simulink model "Beamforming"  (R2019a)
settings: Solver=FixedStepAuto  StartTime=0.0  StopTime=10  RelTol=1e-3
undefined symbols (not defined in the file or in its folder): phased
libraries: dspstat3 x2, phasedtxrxlib x2, phaseddoalib x2
settings Model: Creator=saadn  LastModifiedBy=saadn
settings OptimizationCC: DefaultParameterBehavior=Inlined  UseDivisionForNetSlopeComputation=on  GainParamInheritBuiltInType=on  UseFloatMulNetSlope=on  InlineInvariantSignals=on  PassReuseOutputArgsAs=Individual arguments  ZeroExternalMemoryAtStartup=off  ZeroInternalMemoryAtStartup=off  NoFixptDivByZeroProtection=on  EfficientFloat2IntCast=on  LifeSpan=1  OptimizeBlockOrder=speed  DifferentSizesBufferReuse=on
settings DebuggingCC: ParameterTunabilityLossMsg=error
settings HardwareCC: ProdLongLongMode=on
settings SFSimCC: MATLABDynamicMemAlloc=off
settings RTWCC: SystemTargetFile=ert.tlc  GenCodeOnly=on  TemplateMakefile=ert_default_tmf  GenerateReport=on  IncludeHyperlinkInReport=on  LaunchReport=on  TargetLang=C++  GenerateTraceInfo=on  GenerateTraceReport=on  GenerateTraceReportSl=on  GenerateTraceReportSf=on  GenerateTraceReportEml=on
settings CodeAppCC: GenerateComments=off  IgnoreCustomStorageClasses=off  OperatorAnnotations=on  SimulinkDataObjDesc=on  SFDataObjDesc=on  CustomSymbolStrGlobalVar=rt$N$M  CustomSymbolStrType=$N$M  CustomSymbolStrFcn=$N$M$F  CustomSymbolStrMacro=$N$M  InsertBlockDesc=on
settings ERTTargetCC: TargetLangStandard=C++03 (ISO)  GenerateSampleERTMain=on  IncludeMdlTerminateFcn=off  CombineSignalStateStructs=on  MultiInstanceERTCode=on  CodeInterfacePackaging=C++ class  SupportContinuousTime=on  InlinedParameterPlacement=NonHierarchical  RootIOFormat=Structure reference  ERTCustomFileTemplate=example_file_process.tlc  ERTFilePackagingFormat=CompactWithDataFile

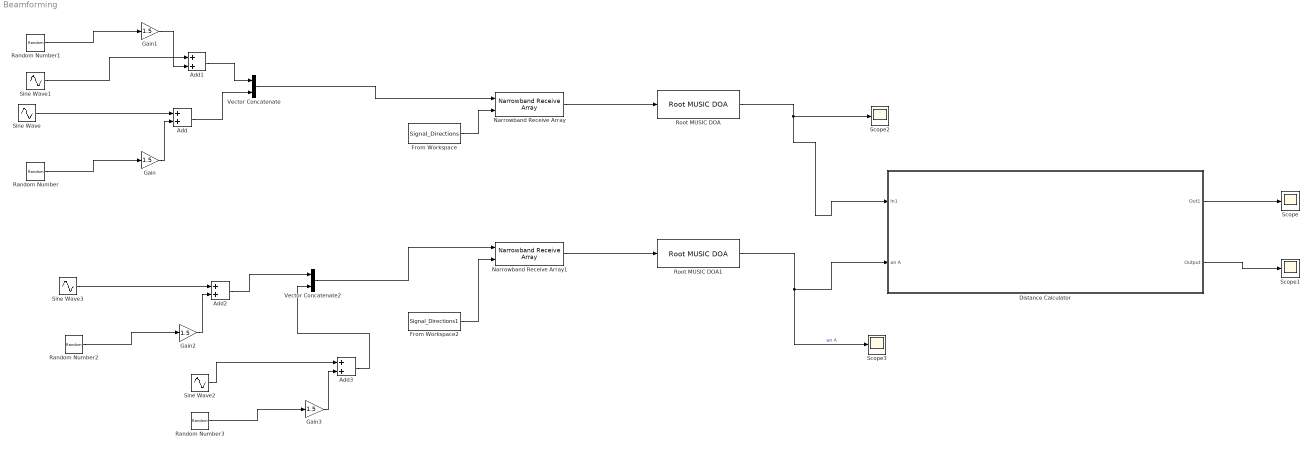
== system Beamforming ==
  Add{,1..3} (4 alike) : Sum
  "Distance Calculator " : Subsystem
  From Workspace : FromWorkspace  VariableName=Signal_Directions  SampleTime=1
  From Workspace2 : FromWorkspace  VariableName=Signal_Directions1  SampleTime=1
  Gain{,1..3} (4 alike) : Gain  Gain=1.5
  Narrowband Receive Array : phasedtxrxlib/Narrowband Receive Array  PropagationSpeed=343  OperatingFrequency=250  Wavefront=Plane  SensorGainMeasure=dB  Polarization=None  WeightsInputPort=off  SimulateUsing=Interpreted execution  Sensor=phased.ULA('Element',phased.IsotropicAntennaElement('FrequencyRange',[ 50, 500 ]),'NumElements',2,'ElementSpacing',0.1)
      settings: SourceProductName=Phased Array System Toolbox  SourceProductBaseCode=AR
  Narrowband Receive Array1 : phasedtxrxlib/Narrowband Receive Array  PropagationSpeed=343  OperatingFrequency=250  Wavefront=Plane  SensorGainMeasure=dB  Polarization=None  WeightsInputPort=off  SimulateUsing=Interpreted execution  Sensor=phased.ULA('Element',phased.IsotropicAntennaElement('FrequencyRange',[ 50, 500 ]),'NumElements',2,'ElementSpacing',0.1)
      settings: SourceProductName=Phased Array System Toolbox  SourceProductBaseCode=AR
  Random Number{,1..3} (4 alike) : RandomNumber  Variance=0.25  SampleTime=0
  Root MUSIC DOA : phaseddoalib/Root MUSIC DOA  PropagationSpeed=343  OperatingFrequency=250  NumSignalsSource=Property  NumSignalsMethod=AIC  NumSignals=1  ForwardBackwardAveraging=off  SpatialSmoothing=0  SimulateUsing=Interpreted execution  SensorArray=phased.ULA('Element',phased.IsotropicAntennaElement('FrequencyRange',[ 50, 500 ]),'NumElements',2,'ElementSpacing',0.1)
      settings: SourceProductName=Phased Array System Toolbox  SourceProductBaseCode=AR
  Root MUSIC DOA1 : phaseddoalib/Root MUSIC DOA  PropagationSpeed=343  OperatingFrequency=250  NumSignalsSource=Property  NumSignalsMethod=AIC  NumSignals=1  ForwardBackwardAveraging=off  SpatialSmoothing=0  SimulateUsing=Interpreted execution  SensorArray=phased.ULA('Element',phased.IsotropicAntennaElement('FrequencyRange',[ 50, 500 ]),'NumElements',2,'ElementSpacing',0.1)
      settings: SourceProductName=Phased Array System Toolbox  SourceProductBaseCode=AR
  Scope{,1..3} (4 alike) : Scope
  Sine Wave : Sin  Amplitude=0.8  Frequency=1067  SampleTime=0
  Sine Wave1 : Sin  Frequency=1067  SampleTime=0
  Sine Wave2 : Sin  Amplitude=0.7  Frequency=1067  SampleTime=0
  Sine Wave3 : Sin  Amplitude=0.8  Frequency=1067  SampleTime=0
  Vector Concatenate : Concatenate
  Vector Concatenate2 : Concatenate
  wires:
  From Workspace/1 -> Narrowband Receive Array/2
  Sine Wave1/1 -> Add1/1
  Sine Wave/1 -> Add/1
  Vector Concatenate2/1 -> Narrowband Receive Array1/1
  From Workspace2/1 -> Narrowband Receive Array1/2
  Root MUSIC DOA/1 -> "Distance Calculator "/1(In1), Scope2/1
  Root MUSIC DOA1/1 -> Scope3/1, "Distance Calculator "/2(an A)  "an A"
  "Distance Calculator "/1(Out1) -> Scope/1
  "Distance Calculator "/2(Output) -> Scope1/1
  Gain/1 -> Add/2
  Random Number/1 -> Gain/1
  Random Number1/1 -> Gain1/1
  Gain1/1 -> Add1/2
  Add/1 -> Vector Concatenate/2
  Add1/1 -> Vector Concatenate/1
  Vector Concatenate/1 -> Narrowband Receive Array/1
  Sine Wave3/1 -> Add2/1
  Random Number2/1 -> Gain2/1
  Gain2/1 -> Add2/2
  Add2/1 -> Vector Concatenate2/1
  Sine Wave2/1 -> Add3/1
  Random Number3/1 -> Gain3/1
  Gain3/1 -> Add3/2
  Add3/1 -> Vector Concatenate2/2
  Narrowband Receive Array/1 -> Root MUSIC DOA/1
  Narrowband Receive Array1/1 -> Root MUSIC DOA1/1

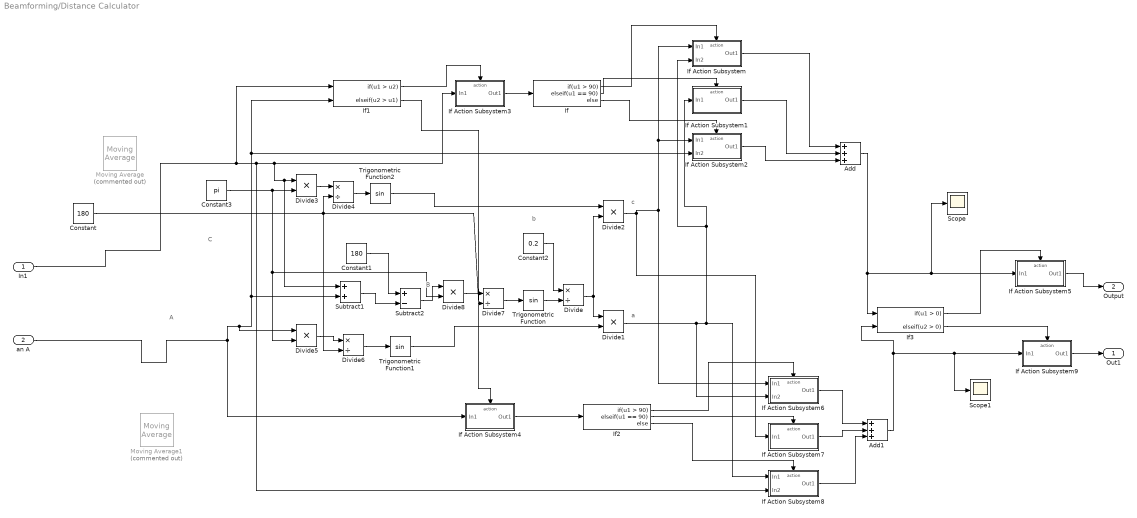
== system Beamforming/Distance Calculator  ==
  note: c
  note: b
  note: a
  note: B
  note: C
  note: A
  In1 : Inport
  an A : Inport  Port=2
  Add : Sum  Inputs=+++
  Add1 : Sum  Inputs=+++
  Constant : Constant  Value=180
  Constant1 : Constant  Value=180
  Constant2 : Constant  Value=0.2
  Constant3 : Constant  Value=pi
  Divide{,4,6..7} (4 alike) : Product  Inputs=*/
  Divide{1..3,5,8} (5 alike) : Product  Inputs=**
  If : If  IfExpression=u1 > 90  ElseIfExpressions=u1 == 90
  If Action Subsystem : Subsystem  TreatAsAtomicUnit=on
  If Action Subsystem1 : Subsystem  TreatAsAtomicUnit=on
  If Action Subsystem2 : Subsystem  TreatAsAtomicUnit=on
  If Action Subsystem3 : Subsystem  TreatAsAtomicUnit=on
  If Action Subsystem4 : Subsystem  TreatAsAtomicUnit=on
  If Action Subsystem5 : Subsystem  TreatAsAtomicUnit=on
  If Action Subsystem6 : Subsystem  TreatAsAtomicUnit=on
  If Action Subsystem7 : Subsystem  TreatAsAtomicUnit=on
  If Action Subsystem8 : Subsystem  TreatAsAtomicUnit=on
  If Action Subsystem9 : Subsystem  TreatAsAtomicUnit=on
  If1 : If  NumInputs=2  IfExpression=u1 > u2  ElseIfExpressions=u2 > u1  ShowElse=off
  If2 : If  IfExpression=u1 > 90  ElseIfExpressions=u1 == 90
  If3 : If  NumInputs=2  ElseIfExpressions=u2 > 0  ShowElse=off
  Moving Average : dspstat3/Moving Average  Commented=on  Method=Sliding window  ForgettingFactorPort=off  SpecifyWindowLength=on  WindowLength=3  ForgettingFactor=0.9  SimulateUsing=Interpreted execution
  Moving Average1 : dspstat3/Moving Average  Commented=on  Method=Sliding window  ForgettingFactorPort=off  SpecifyWindowLength=on  WindowLength=3  ForgettingFactor=0.9  SimulateUsing=Interpreted execution
  Scope : Scope
  Scope1 : Scope
  Subtract1 : Sum
  Subtract2 : Sum  Inputs=+-
  Trigonometric Function : Trigonometry
  Trigonometric Function1 : Trigonometry  OutputSignalType=real
  Trigonometric Function2 : Trigonometry  OutputSignalType=real
  Out1 : Outport
  Output : Outport  Port=2
  wires:
  If/2 -> If Action Subsystem1/Action
  Divide1/1 -> If Action Subsystem6/2(In2), If Action Subsystem8/1(In1), If Action Subsystem1/1(In1), If Action Subsystem/2(In2)
  Divide/1 -> Divide1/1, Divide2/2
  Constant/1 -> Divide7/2, Divide6/2, Divide4/2
  If Action Subsystem4/1(Out1) -> If2/1
  Constant3/1 -> Divide8/2, Divide5/2, Divide3/2
  If2/3 -> If Action Subsystem8/Action
  Trigonometric Function1/1 -> Divide1/2
  If1/1 -> If Action Subsystem3/Action
  Divide2/1 -> If Action Subsystem6/1(In1), If Action Subsystem2/1(In1), If Action Subsystem/1(In1), If Action Subsystem7/1(In1)
  If2/1 -> If Action Subsystem6/Action
  Constant2/1 -> Divide/1
  Trigonometric Function2/1 -> Divide2/1
  Divide7/1 -> Trigonometric Function/1
  Divide8/1 -> Divide7/1
  Subtract2/1 -> Divide8/1
  Trigonometric Function/1 -> Divide/2
  Subtract1/1 -> Subtract2/2
  Divide4/1 -> Trigonometric Function2/1
  If Action Subsystem7/1(Out1) -> Add1/2
  If Action Subsystem1/1(Out1) -> Add/2
  Divide6/1 -> Trigonometric Function1/1
  If Action Subsystem3/1(Out1) -> If/1
  If1/2 -> If Action Subsystem4/Action
  Add/1 -> Scope/1, If Action Subsystem5/1(In1), If3/1
  If/3 -> If Action Subsystem2/Action
  Constant1/1 -> Subtract2/1
  If Action Subsystem8/1(Out1) -> Add1/3
  If Action Subsystem6/1(Out1) -> Add1/1
  If Action Subsystem/1(Out1) -> Add/1
  If/1 -> If Action Subsystem/Action
  If Action Subsystem2/1(Out1) -> Add/3
  If2/2 -> If Action Subsystem7/Action
  Add1/1 -> Scope1/1, If Action Subsystem9/1(In1), If3/2
  Divide3/1 -> Divide4/1
  Divide5/1 -> Divide6/1
  an A/1 -> If1/2, If Action Subsystem2/2(In2), Subtract1/2, Divide5/1, If Action Subsystem4/1(In1)
  In1/1 -> If1/1, If Action Subsystem8/2(In2), Subtract1/1, Divide3/1, If Action Subsystem3/1(In1)
  If3/1 -> If Action Subsystem5/Action
  If3/2 -> If Action Subsystem9/Action
  If Action Subsystem5/1(Out1) -> Output/1
  If Action Subsystem9/1(Out1) -> Out1/1

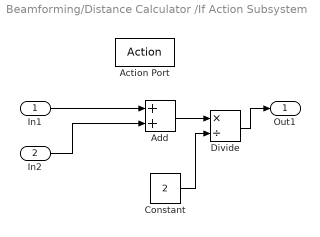
== system Beamforming/Distance Calculator /If Action Subsystem ==
  In1 : Inport
  In2 : Inport  Port=2
  Action Port : ActionPort  InitializeStates=reset  ActionPortLabel=if(u1 > 90)
  Add : Sum
  Constant : Constant  Value=2
  Divide : Product  Inputs=*/
  Out1 : Outport
  wires:
  In1/1 -> Add/1
  In2/1 -> Add/2
  Add/1 -> Divide/1
  Constant/1 -> Divide/2
  Divide/1 -> Out1/1

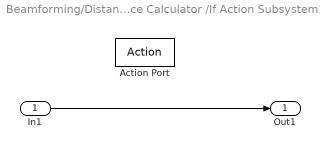
== system Beamforming/Distance Calculator /If Action Subsystem1 ==
  In1 : Inport
  Action Port : ActionPort  InitializeStates=reset  ActionPortLabel=elseif(u1 == 90)
  Out1 : Outport
  wires:
  In1/1 -> Out1/1

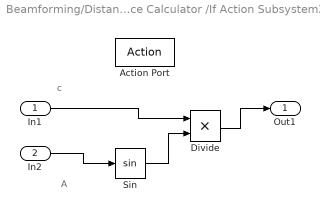
== system Beamforming/Distance Calculator /If Action Subsystem2 ==
  note: A
  note: c
  In1 : Inport
  In2 : Inport  Port=2
  Action Port : ActionPort  InitializeStates=reset  ActionPortLabel=else
  Divide : Product  Inputs=**
  Sin : Trigonometry
  Out1 : Outport
  wires:
  In1/1 -> Divide/1
  In2/1 -> Sin/1
  Sin/1 -> Divide/2
  Divide/1 -> Out1/1

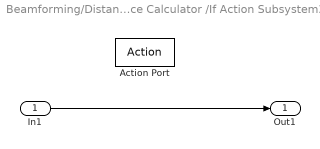
== system Beamforming/Distance Calculator /If Action Subsystem3 ==
  In1 : Inport
  Action Port : ActionPort  InitializeStates=reset  ActionPortLabel=if(u1 > u2)
  Out1 : Outport
  wires:
  In1/1 -> Out1/1

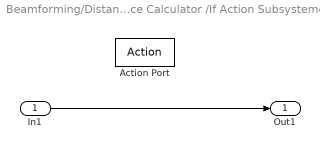
== system Beamforming/Distance Calculator /If Action Subsystem4 ==
  In1 : Inport
  Action Port : ActionPort  InitializeStates=reset  ActionPortLabel=elseif(u2 > u1)
  Out1 : Outport
  wires:
  In1/1 -> Out1/1

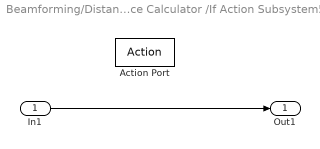
== system Beamforming/Distance Calculator /If Action Subsystem5 ==
  In1 : Inport
  Action Port : ActionPort  ActionPortLabel=if(u1 > 0)
  Out1 : Outport
  wires:
  In1/1 -> Out1/1

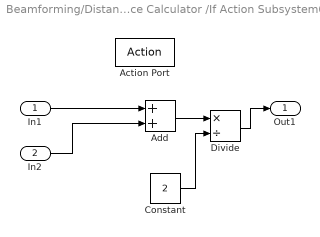
== system Beamforming/Distance Calculator /If Action Subsystem6 ==
  In1 : Inport
  In2 : Inport  Port=2
  Action Port : ActionPort  InitializeStates=reset  ActionPortLabel=if(u1 > 90)
  Add : Sum
  Constant : Constant  Value=2
  Divide : Product  Inputs=*/
  Out1 : Outport
  wires:
  In1/1 -> Add/1
  In2/1 -> Add/2
  Add/1 -> Divide/1
  Constant/1 -> Divide/2
  Divide/1 -> Out1/1

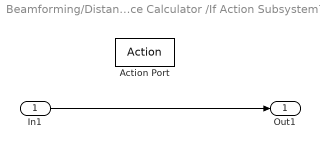
== system Beamforming/Distance Calculator /If Action Subsystem7 ==
  In1 : Inport
  Action Port : ActionPort  InitializeStates=reset  ActionPortLabel=elseif(u1 == 90)
  Out1 : Outport
  wires:
  In1/1 -> Out1/1

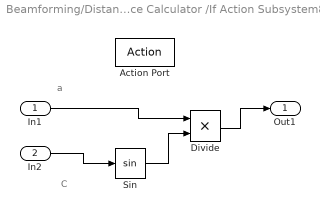
== system Beamforming/Distance Calculator /If Action Subsystem8 ==
  note: C
  note: a
  In1 : Inport
  In2 : Inport  Port=2
  Action Port : ActionPort  InitializeStates=reset  ActionPortLabel=else
  Divide : Product  Inputs=**
  Sin : Trigonometry
  Out1 : Outport
  wires:
  In1/1 -> Divide/1
  In2/1 -> Sin/1
  Sin/1 -> Divide/2
  Divide/1 -> Out1/1

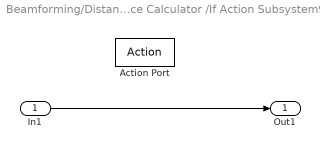
== system Beamforming/Distance Calculator /If Action Subsystem9 ==
  In1 : Inport
  Action Port : ActionPort  ActionPortLabel=elseif(u2 > 0)
  Out1 : Outport
  wires:
  In1/1 -> Out1/1
